simulink model "OCRmodel_2012a_Spring2022"  (R2020b)
settings: Solver=FixedStepDiscrete  StartTime=0.0  StopTime=0.2  FixedStep=50e-6  RelTol=1e-3
libraries: powerlib x12, dspstat3 x2
settings Model: Creator=mishr  LastModifiedBy=Kuldip
settings DataIOCC: SaveFormat=StructureWithTime  ReturnWorkspaceOutputs=off
settings OptimizationCC: LifeSpan=inf
settings DebuggingCC: FcnCallInpInsideContextMsg=warning  SFExecutionAtInitializationDiag=none  ArithmeticOperatorsInVariantConditions=warning
settings HardwareCC: ProdBitPerSizeT=32  ProdBitPerPtrDiffT=32  ProdWordSize=32  ProdHWDeviceType=Specified
settings SFSimCC: SimUseLocalCustomCode=off  CustomCodeUndefinedFunction=UseInterfaceOnly
settings RTWCC: RTWUseLocalCustomCode=off
settings CodeAppCC: StateflowObjectComments=on
settings SimscapeCC: SimscapeNormalizeSystem=off

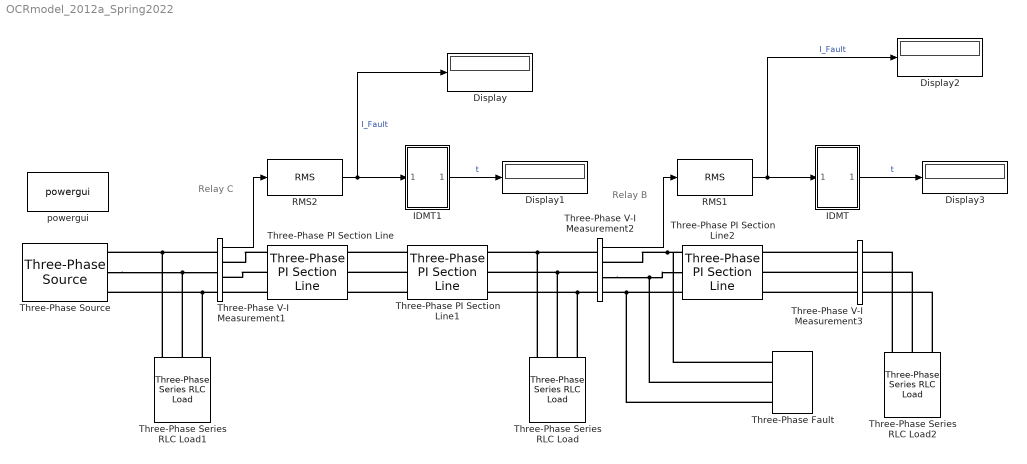
== system OCRmodel_2012a_Spring2022 ==
  note: Relay C
  note: Relay B
  Display{,1..3} (4 alike) : Display
  IDMT : Subsystem
  IDMT1 : Subsystem
  RMS1 : dspstat3/RMS  run=off  directionMode=Each column  dimension=1  InputProcessing=Columns as channels (frame based)  reset_popup=None
  RMS2 : dspstat3/RMS  run=off  directionMode=Each column  dimension=1  InputProcessing=Columns as channels (frame based)  reset_popup=None
  Three-Phase PI Section Line : powerlib/Elements/Three-Phase PI Section Line  LConnTagsString=a|b|c  RConnTagsString=A|B|C  Length=5  Frequency=60  Resistances=[ 3.89 3.89*2]/10  Inductances=[2.63 2.63*2]/(10*2*3.14*60)  Capacitances=[12.74e-9 7.751e-9]
  Three-Phase PI Section Line1 : powerlib/Elements/Three-Phase PI Section Line  LConnTagsString=a|b|c  RConnTagsString=A|B|C  Length=5  Frequency=60  Resistances=[ 3.89 3.89*2]/10  Inductances=[2.63 2.63*2]/(10*2*3.14*60)  Capacitances=[12.74e-9 7.751e-9]
  Three-Phase PI Section Line2 : powerlib/Elements/Three-Phase PI Section Line  LConnTagsString=a|b|c  RConnTagsString=A|B|C  Length=5  Frequency=60  Resistances=[ 3.89 3.89*2]/10  Inductances=[2.63 2.63*2]/(10*2*3.14*60)  Capacitances=[12.74e-9 7.751e-9]
  Three-Phase Series RLC Load : powerlib/Elements/Three-Phase Series RLC Load  LConnTagsString=A|B|C  Configuration=Y (grounded)  NominalVoltage=12.47e3  Vabc=[1e3 1e3 1e3]  Vabcp=[1e3 1e3 1e3]  NominalFrequency=60  UnbalancedPower=off  ActivePower=0.89e6  InductivePower=0.45e6  CapacitivePower=0  Pabc=[10e3 9e3 11e3]  QLabc=[100 90 110]  QCabc=[100 90 110]  Pabcp=[10e3 9e3 11e3]  QLabcp=[100 90 110]  QCabcp=[100 90 110]  Measurements=None  LoadType=constant Z
  Three-Phase Series RLC Load1 : powerlib/Elements/Three-Phase Series RLC Load  LConnTagsString=A|B|C  Configuration=Y (grounded)  NominalVoltage=12.47e3  Vabc=[1e3 1e3 1e3]  Vabcp=[1e3 1e3 1e3]  NominalFrequency=60  UnbalancedPower=off  ActivePower=2.02e6  InductivePower=0.95e6  CapacitivePower=0  Pabc=[10e3 9e3 11e3]  QLabc=[100 90 110]  QCabc=[100 90 110]  Pabcp=[10e3 9e3 11e3]  QLabcp=[100 90 110]  QCabcp=[100 90 110]  Measurements=None  LoadType=constant Z
  Three-Phase Series RLC Load2 : powerlib/Elements/Three-Phase Series RLC Load  LConnTagsString=A|B|C  Configuration=Y (grounded)  NominalVoltage=12.47e3  Vabc=[1e3 1e3 1e3]  Vabcp=[1e3 1e3 1e3]  NominalFrequency=60  UnbalancedPower=off  ActivePower=0.82e6  InductivePower=0.5e6  CapacitivePower=0  Pabc=[10e3 9e3 11e3]  QLabc=[100 90 110]  QCabc=[100 90 110]  Pabcp=[10e3 9e3 11e3]  QLabcp=[100 90 110]  QCabcp=[100 90 110]  Measurements=None  LoadType=constant Z
  Three-Phase V-I Measurement1 : powerlib/Measurements/Three-Phase V-I Measurement  VoltageMeasurement=phase-to-ground  SetLabelV=on  LabelV=Vabc_C  Vpu=off  VpuLL=off  CurrentMeasurement=yes  SetLabelI=off  LabelI=Iabc  Ipu=off  Pbase=100e6  Vbase=500e3  OutputType=Complex  PhasorSimulation=off  PSBequivalent=0
  Three-Phase V-I Measurement2 : powerlib/Measurements/Three-Phase V-I Measurement  VoltageMeasurement=phase-to-ground  SetLabelV=on  LabelV=Vabc_B  Vpu=off  VpuLL=off  CurrentMeasurement=yes  SetLabelI=off  LabelI=Iabc  Ipu=off  Pbase=100e6  Vbase=500e3  OutputType=Complex  PhasorSimulation=off  PSBequivalent=0
  Three-Phase V-I Measurement3 : powerlib/Measurements/Three-Phase V-I Measurement  VoltageMeasurement=phase-to-ground  SetLabelV=on  LabelV=Vabc_A  Vpu=off  VpuLL=off  CurrentMeasurement=yes  SetLabelI=on  LabelI=Iabc_A  Ipu=off  Pbase=100e6  Vbase=500e3  OutputType=Complex  PhasorSimulation=off  PSBequivalent=0
  Three-Phase Fault : powerlib/Elements/Three-Phase Fault  InitialStates=0  FaultA=on  FaultB=off  FaultC=off  GroundFault=on  SwitchTimes=[0.1]  External=off  SwitchStatus=NaN  FaultResistance=9  GroundResistance=0.01  SnubberResistance=1e6  SnubberCapacitance=inf  Measurements=None
  Three-Phase Source : powerlib/Electrical Sources/Three-Phase Source  InternalConnection=Yg  VoltagePhases=off  Voltage=12.47e3  PhaseAngle=0  Voltage_phases=[25e3 25e3 25e3]/sqrt(3)  PhaseAngles_phases=[0 -120 +120]  Frequency=60  NonIdealSource=on  SpecifyImpedance=on  Resistance=0.8929  Inductance=16.58e-3  ShortCircuitLevel=50e6  BaseVoltage=12.47e3  XRratio=10  BusType=swing  Pref=10e3  Qref=0  Prefabc=[10e3, 10e3, 10e3]  Qrefabc=[0, 0, 0]  Qmin=-inf  Qmax=inf
  powergui : powerlib/powergui  Priority=1  SimulationMode=Discrete  SampleTime=50e-6  frequency=60  Iterations=50  frequencyindice=60  Pbase=100e6  ErrMax=1e-4  UnitsV=kV  UnitsW=MW  buscounter=0  FunctionMessages=off  echomessages=off  EnableUseOfTLC=off  CurrentSourceSwitches=off  DisableSnubberDevices=off  DisableRonSwitches=off  DisableVfSwitches=off  DisplayEquations=off  AutomaticDiscreteSolvers=off  SolverType=Tustin/Backward Euler (TBE)  Interpol=off  ExternalGateDelay=off  methode=off  Ts=100  x0status=blocks  SPID=on  SwTol=0  HookPort=off  NonlinearTolerance=1e-4  nMaxIteration=100  ContinueOnMaxIteration=off  RestoreLinks=warning  ResistiveCurrentMeasurement=off  Frange=[0:2:500]  Ylog=off  Xlog=on  ShowGrid=off  save=off  variable=ZData  structure=0  ZoomFFT=off  StartTime=0.0  cycles=1  DisplayStyle=1  fundamental=60  FreqAxis=off  MaxFrequency=1000  frequencyindicesteady=1  RmsSteady=1  display=off
  wires:
  Three-Phase V-I Measurement2/1 -> RMS1/1
  Three-Phase V-I Measurement1/1 -> RMS2/1
  RMS1/1 -> Display2/1, IDMT/1(In1)  "I_Fault"
  IDMT/1(Out1) -> Display3/1  "t"
  RMS2/1 -> Display/1, IDMT1/1(In1)  "I_Fault"
  IDMT1/1(Out1) -> Display1/1  "t"
  connections:
  Three-Phase V-I Measurement1/LConn1 -- Three-Phase Series RLC Load1/LConn1 -- Three-Phase Source/RConn1
  Three-Phase Source/RConn2 -- Three-Phase Series RLC Load1/LConn2 -- Three-Phase V-I Measurement1/LConn2
  Three-Phase V-I Measurement1/LConn3 -- Three-Phase Series RLC Load1/LConn3 -- Three-Phase Source/RConn3
  Three-Phase PI Section Line/LConn1 -- Three-Phase V-I Measurement1/RConn1
  Three-Phase PI Section Line/LConn2 -- Three-Phase V-I Measurement1/RConn2
  Three-Phase PI Section Line/LConn3 -- Three-Phase V-I Measurement1/RConn3
  Three-Phase PI Section Line1/LConn1 -- Three-Phase PI Section Line/RConn1
  Three-Phase PI Section Line1/LConn2 -- Three-Phase PI Section Line/RConn2
  Three-Phase PI Section Line1/LConn3 -- Three-Phase PI Section Line/RConn3
  Three-Phase V-I Measurement2/LConn1 -- Three-Phase Series RLC Load/LConn1 -- Three-Phase PI Section Line1/RConn1
  Three-Phase V-I Measurement2/LConn2 -- Three-Phase Series RLC Load/LConn2 -- Three-Phase PI Section Line1/RConn2
  Three-Phase V-I Measurement2/LConn3 -- Three-Phase Series RLC Load/LConn3 -- Three-Phase PI Section Line1/RConn3
  Three-Phase PI Section Line2/LConn1 -- Three-Phase V-I Measurement2/RConn1 -- Three-Phase Fault/LConn1
  Three-Phase V-I Measurement2/RConn2 -- Three-Phase Fault/LConn2 -- Three-Phase PI Section Line2/LConn2
  Three-Phase PI Section Line2/LConn3 -- Three-Phase Fault/LConn3 -- Three-Phase V-I Measurement2/RConn3
  Three-Phase V-I Measurement3/LConn1 -- Three-Phase PI Section Line2/RConn1
  Three-Phase V-I Measurement3/LConn2 -- Three-Phase PI Section Line2/RConn2
  Three-Phase V-I Measurement3/LConn3 -- Three-Phase PI Section Line2/RConn3
  Three-Phase Series RLC Load2/LConn1 -- Three-Phase V-I Measurement3/RConn1
  Three-Phase Series RLC Load2/LConn2 -- Three-Phase V-I Measurement3/RConn2
  Three-Phase Series RLC Load2/LConn3 -- Three-Phase V-I Measurement3/RConn3

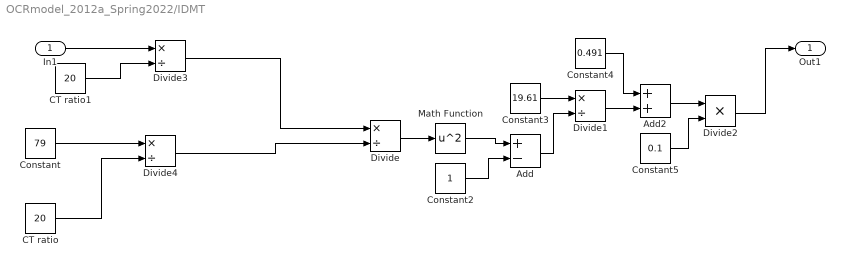
== system OCRmodel_2012a_Spring2022/IDMT ==
  In1 : Inport
  Add : Sum  Inputs=+-
  Add2 : Sum
  CT ratio : Constant  Value=20
  CT ratio1 : Constant  Value=20
  Constant : Constant  Value=79
  Constant2 : Constant
  Constant3 : Constant  Value=19.61
  Constant4 : Constant  Value=0.491
  Constant5 : Constant  Value=0.1
  Divide{,1,3..4} (4 alike) : Product  Inputs=*/
  Divide2 : Product  Inputs=**
  Math Function : Math  Operator=square  SignedPower=on  SaturateOnIntegerOverflow=on
  Out1 : Outport
  wires:
  Divide1/1 -> Add2/2
  Constant3/1 -> Divide1/1
  Add2/1 -> Divide2/1
  Constant5/1 -> Divide2/2
  Divide/1 -> Math Function/1
  Math Function/1 -> Add/1
  Add/1 -> Divide1/2
  Constant4/1 -> Add2/1
  Constant2/1 -> Add/2
  Divide2/1 -> Out1/1
  Constant/1 -> Divide4/1
  CT ratio/1 -> Divide4/2
  CT ratio1/1 -> Divide3/2
  Divide3/1 -> Divide/1
  Divide4/1 -> Divide/2
  In1/1 -> Divide3/1

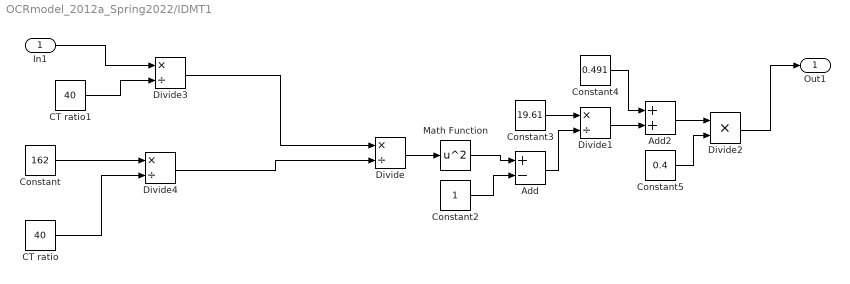
== system OCRmodel_2012a_Spring2022/IDMT1 ==
  In1 : Inport
  Add : Sum  Inputs=+-
  Add2 : Sum
  CT ratio : Constant  Value=40
  CT ratio1 : Constant  Value=40
  Constant : Constant  Value=162
  Constant2 : Constant
  Constant3 : Constant  Value=19.61
  Constant4 : Constant  Value=0.491
  Constant5 : Constant  Value=0.4
  Divide{,1,3..4} (4 alike) : Product  Inputs=*/
  Divide2 : Product  Inputs=**
  Math Function : Math  Operator=square  SignedPower=on  SaturateOnIntegerOverflow=on
  Out1 : Outport
  wires:
  Divide1/1 -> Add2/2
  Constant3/1 -> Divide1/1
  Add2/1 -> Divide2/1
  Constant5/1 -> Divide2/2
  Divide/1 -> Math Function/1
  Math Function/1 -> Add/1
  Add/1 -> Divide1/2
  Constant4/1 -> Add2/1
  Constant2/1 -> Add/2
  Divide2/1 -> Out1/1
  Constant/1 -> Divide4/1
  CT ratio/1 -> Divide4/2
  In1/1 -> Divide3/1
  CT ratio1/1 -> Divide3/2
  Divide3/1 -> Divide/1
  Divide4/1 -> Divide/2
